simulink model "simple"  (Simulink 4.00)
settings: Solver=ode45  StartTime=0.0  StopTime=10.0  RelTol=1e-3
libraries: simulink3 x1, truetime x1
settings Model: Creator=anton  LastModifiedBy=anton  ExtModeAutoUpdateStatusClock=off

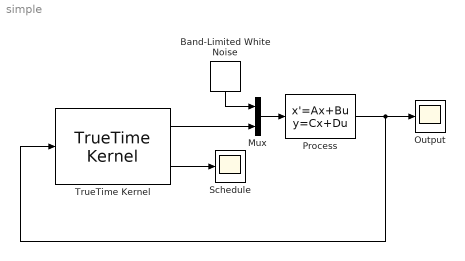
== system simple ==
  Band-Limited White Noise : simulink3/Sources/Band-Limited White Noise  Orientation=down  Cov=[0.1]  Ts=0.1  seed=[23341]
  Mux : Mux  Inputs=2
  Output : Scope
      settings: TimeRange=auto  YMin=-5  YMax=5  SaveToWorkspace=off  LimitDataPoints=on  MaxDataPoints=5000
  Process : StateSpace  A=1  B=1  C=1  D=1  X0=0  AbsoluteTolerance=auto  Realization=auto
  Schedule : Scope
      settings: TimeRange=auto  YMin=-5  YMax=5  SaveToWorkspace=off  SaveName=ScopeData  LimitDataPoints=on  MaxDataPoints=5000
  TrueTime Kernel : truetime/TrueTime Kernel  sfun=node_init  args=[]  ninputsoutputs=[1 1]  ntriggers=0  nwnodenbr=[]  clockoffsetdrift=[0 0]  schedoutput=on  monitorsoutput=off  battery=off  poweroutput=off
  wires:
  TrueTime Kernel/2 -> Schedule/1
  Process/1 -> TrueTime Kernel/1, Output/1
  TrueTime Kernel/1 -> Mux/2
  Mux/1 -> Process/1
  Band-Limited White Noise/1 -> Mux/1
